simulink model "silnik_wzor"  (Simulink 10.3)
settings: Solver=ode3  StartTime=0.0  StopTime=1  FixedStep=0.001  RelTol=1e-3  EnableMultiTasking=on
InitFcn:
  | % Parametry obiektu
  | R = 3;
  | L = 0.05;
  | kfi = 2.23;
  | J = 0.11;
values from neighbouring files (symbols this model uses):
  Lo = acker(A', C', [-w0, -w0])    [lab04z1.m]
settings Model: Creator=Jacek  LastModifiedBy=AgraWoodAdmin
settings DataIOCC: LimitDataPoints=on  SignalLoggingSaveFormat=Dataset
settings OptimizationCC: ExpressionDepthLimit=128
settings DebuggingCC: UnderspecifiedInitializationDetection=Simplified  MergeDetectMultiDrivingBlocksExec=error  SolverPrmCheckMsg=warning  FcnCallInpInsideContextMsg=error  StateNameClashWarn=none
settings GRTTargetCC: CombineOutputUpdateFcns=on  GRTInterface=off
settings ConfigComp: CovSFcnEnable=off

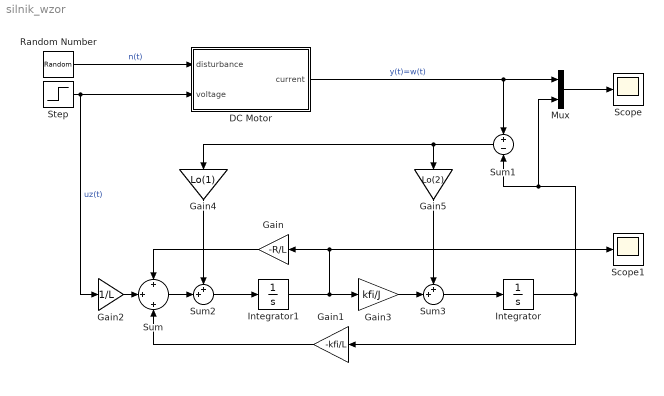
== system silnik_wzor ==
  DC Motor : Subsystem
  Gain : Gain  Gain=-R/L
  Gain1 : Gain  Gain=-kfi/L
  Gain2 : Gain  Gain=1/L
  Gain3 : Gain  Gain=kfi/J
  Gain4 : Gain  Gain=Lo(1)
  Gain5 : Gain  Gain=Lo(2)
  Integrator : Integrator  InitialCondition=60
  Integrator1 : Integrator
  Mux : Mux  Inputs=2
  Random Number : RandomNumber  Variance=10
  Scope : Scope
  Scope1 : Scope
  Step : Step  Time=0  After=300  SampleTime=0
  Sum : Sum  Inputs=+|+|+
  Sum1 : Sum  Inputs=+|-
  Sum2 : Sum  Inputs=++|
  Sum3 : Sum  Inputs=++|
  wires:
  Random Number/1 -> DC Motor/1(disturbance)  "n(t)"
  Step/1 -> Gain2/1, DC Motor/2(voltage)  "uz(t)"
  DC Motor/1(current) -> Sum1/1, Mux/1  "y(t)=w(t)"
  Integrator1/1 -> Gain/1, Scope1/1, Gain3/1
  Gain/1 -> Sum/1
  Integrator/1 -> Mux/2, Sum1/2, Gain1/1
  Gain1/1 -> Sum/3
  Gain2/1 -> Sum/2
  Mux/1 -> Scope/1
  Sum1/1 -> Gain4/1, Gain5/1
  Sum2/1 -> Integrator1/1
  Sum3/1 -> Integrator/1
  Gain3/1 -> Sum3/2
  Gain5/1 -> Sum3/1
  Sum/1 -> Sum2/2
  Gain4/1 -> Sum2/1

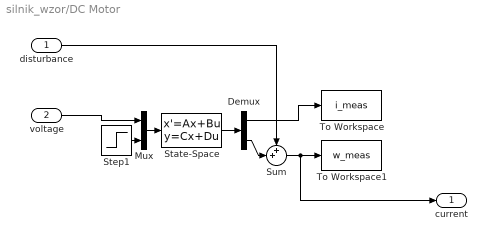
== system silnik_wzor/DC Motor ==
  disturbance : Inport
  voltage : Inport  Port=2
  Demux : Demux  Outputs=2
  Mux : Mux  Inputs=2
  State-Space : StateSpace  A=[-3/0.05, -2.23/0.05; 2.23/0.11, 0]  B=[1/0.05 0; 0 -1/0.11]  C=[1 0;0 1]  D=[0 0; 0 0]  InitialCondition=[0 ;40]
  Step1 : Step  Time=0.5  After=44.6  SampleTime=0
  Sum : Sum  Inputs=++|
  To Workspace : ToWorkspace  VariableName=i_meas  SampleTime=-1
  To Workspace1 : ToWorkspace  VariableName=w_meas  SampleTime=-1
  current : Outport  VectorParamsAs1DForOutWhenUnconnected=off
  wires:
  Mux/1 -> State-Space/1
  voltage/1 -> Mux/1
  Step1/1 -> Mux/2
  State-Space/1 -> Demux/1
  disturbance/1 -> Sum/1
  Demux/2 -> Sum/2
  Demux/1 -> To Workspace/1
  Sum/1 -> current/1, To Workspace1/1
